simulink model "Reaching"  (R2024b)
settings: Solver=FixedStepDiscrete  StartTime=0.0  StopTime=inf  FixedStep=0.001  RelTol=1e-3
undefined symbols (not defined in the file): get
libraries: vrlib x3, PhanTorque_3Dof_Library_64Bits x1
settings Model: Creator=carlos.aldana  LastModifiedBy=alvinisac
settings SolverCC: AlgebraicLoopSolver=TrustRegion
settings DataIOCC: LimitDataPoints=on  SaveFormat=Array  ReturnWorkspaceOutputs=off
settings OptimizationCC: BlockReduction=off  BooleanDataType=off  LifeSpan=inf
settings DebuggingCC: SaveWithParameterizedLinksMsg=none  UnderspecifiedInitializationDetection=Classic  MergeDetectMultiDrivingBlocksExec=none  SignalResolutionControl=TryResolveAllWithWarning  UnconnectedInputMsg=warning  UnconnectedOutputMsg=warning  UnconnectedLineMsg=warning  AllowSymbolicDim=off  SFUnexpectedBacktrackingDiag=warning  SFNoUnconditionalDefaultTransitionDiag=warning  SFExecutionAtInitializationDiag=none  ArithmeticOperatorsInVariantConditions=warning
settings HardwareCC: ProdBitPerPointer=32  ProdBitPerSizeT=32  ProdBitPerPtrDiffT=32  ProdLargestAtomicFloat=None  ProdIntDivRoundTo=Undefined  ProdEndianess=Unspecified  ProdWordSize=32  ProdHWDeviceType=32-bit Generic  TargetUnknown=on
settings ModelReferenceCC: EnableRefExpFcnMdlSchedulingChecks=on  PropagateSignalLabelsOutOfModel=off
settings SFSimCC: SimUseLocalCustomCode=off  CustomCodeUndefinedFunction=UseInterfaceOnly
settings RTWCC: RTWUseLocalCustomCode=off  GPUComputeCapability=3.5  DLArmComputeVersion=19.05
settings CodeAppCC: StateflowObjectComments=on
settings GRTTargetCC: TargetLangStandard=C89/C90 (ANSI)
settings ConfigComp: CovMetricSettings=dw  CovSaveCumulativeToWorkspaceVar=on  CovSaveSingleToWorkspaceVar=on  CovExternalEMLEnable=off  CovSFcnEnable=off

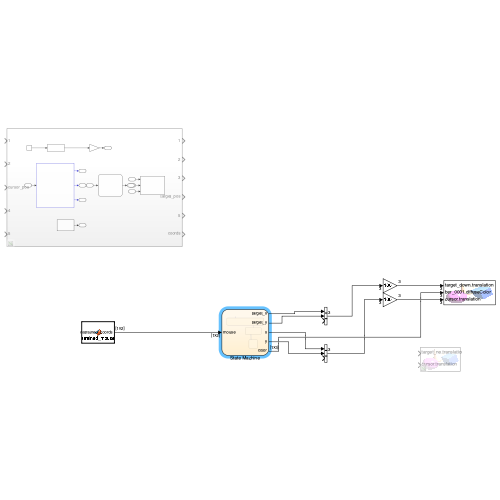
[thumbnail: Simulink's stored preview of the top-level diagram]
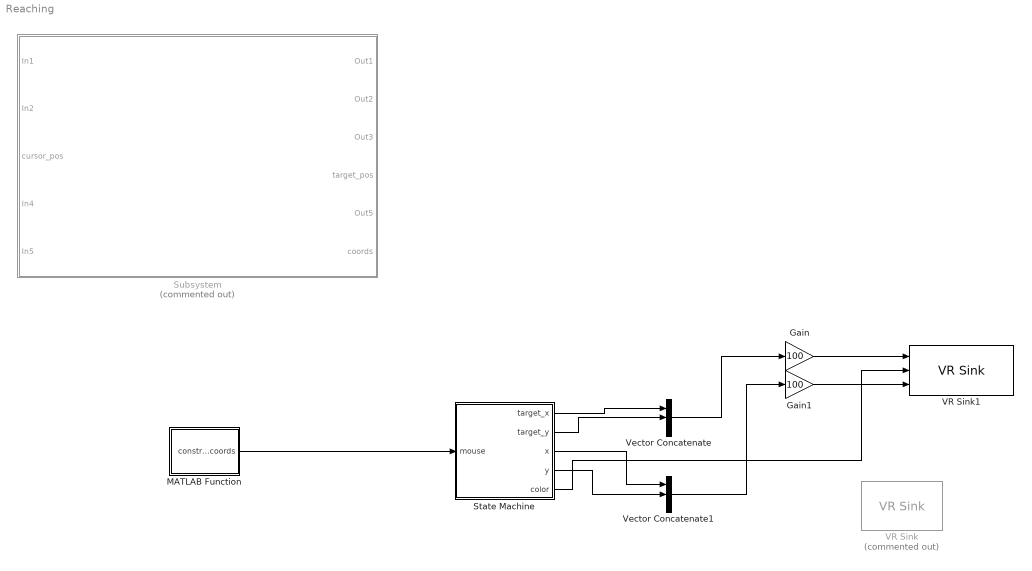
== system Reaching ==
  Gain : Gain  Gain=100
  Gain1 : Gain  Gain=100
  MATLAB Function : MATLAB Function  TreatAsAtomicUnit=on
  State Machine : Stateflow chart  TreatAsAtomicUnit=on
  Subsystem : Subsystem  Commented=on
  VR Sink : vrlib/VR Sink  Commented=on  InstantiateOnLoad=on  SampleTime=0.1  ViewEnable=on  RemoteChange=off  RemoteView=off  FieldsWritten=target_ne.translation.3.1.1.double#cursor.translation.3.1.1.double  WorldFileName=8_palline_color.wrl  AutoView=off  VideoDimensions=[]  AllowVariableSize=off
  VR Sink1 : vrlib/VR Sink  InstantiateOnLoad=on  SampleTime=0.1  ViewEnable=on  RemoteChange=off  RemoteView=off  FieldsWritten=target_down.translation.3.1.1.double#ber_0001.diffuseColor.3.1.1.double#cursor.translation.3.1.1.double  WorldFileName=VR_centerAndTarget.wrl  AutoView=off  VideoDimensions=[]  AllowVariableSize=off  FigureProperties="{'Position', 'Name', 'Viewpoint', 'CameraBound', 'CameraDirection', 'CameraPosition', 'CameraUpVector', 'ZoomFactor', 'Antialiasing', 'Headlight', 'Lighting', 'Sound', 'StatusBar', 'Stereo3D', 'Stereo3DCameraOffset', 'Stereo3DHIT', 'ToolBar', 'Textures', 'Transparency', 'Triad', 'Wireframe', 'NavZones', 'NavMode', 'NavSpeed', 'CaptureFileFormat', 'CaptureFileName', 'Record2DCompressMethod', 'Record2DCompressQuality', 'Record2D', 'Record2DFileName', 'Record2DFPS', 'NavPanel'; [5.0000000000000000e+00   1.0300000000000000e+02   5.7600000000000000e+02   3.5000000000000000e+02], '', '_untitled_1', 'on', [0.0000000000000000e+00   0.0000000000000000e+00  -1.0000000000000000e+00], [0.0000000000000000e+00   0.0000000000000000e+00   0.0000000000000000e+00], [0.0000000000000000e+00   1.0000000000000000e+00   0.0000000000000000e+00], [1.0000000000000000e+00], 'on', 'on', 'on', 'on', 'on', 'off', [1.0000000149011612e-01], [0.0000000000000000e+00], 'on', 'on', 'on', 'none', 'off', 'off', 'fly', 'normal', 'tif', '%f_anim_%n.tif', 'auto', [7.5000000000000000e+01], 'off', '%f_anim_%n.avi', 'auto', 'halfbar'}"
  Vector Concatenate : Concatenate  NumInputs=3
  Vector Concatenate1 : Concatenate  NumInputs=3
  wires:
  MATLAB Function/1(constrained_coords) -> State Machine/1(mouse)
  State Machine/1(target_x) -> Vector Concatenate/1
  State Machine/2(target_y) -> Vector Concatenate/2
  State Machine/4(y) -> Vector Concatenate1/2
  State Machine/3(x) -> Vector Concatenate1/1
  Vector Concatenate1/1 -> Gain1/1
  Vector Concatenate/1 -> Gain/1
  Gain/1 -> VR Sink1/1
  Gain1/1 -> VR Sink1/3
  State Machine/5(color) -> VR Sink1/2

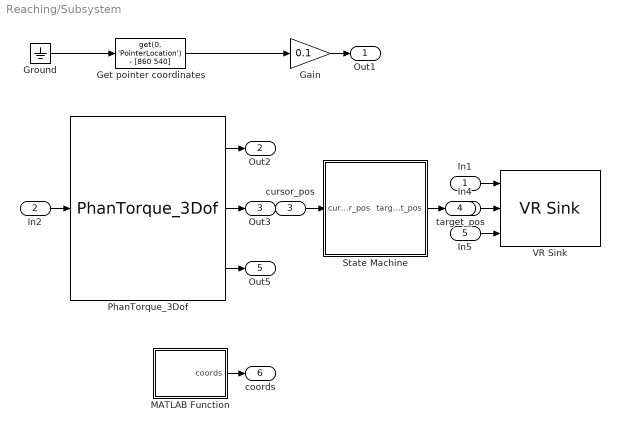
== system Reaching/Subsystem ==
  In1 : Inport
  In2 : Inport  Port=2
  cursor_pos : Inport  Port=3
  In4 : Inport  Port=4
  In5 : Inport  Port=5
  Gain : Gain  Gain=0.1
  Get pointer coordinates : MATLABFcn  MATLABFcn=get(0, 'PointerLocation') - [860 540]  OutputDimensions=2
  Ground : Ground
  MATLAB Function : MATLAB Function  TreatAsAtomicUnit=on
  PhanTorque_3Dof : PhanTorque_3Dof_Library_64Bits/PhanTorque_3Dof  Haptic_Name='Default Device'
  State Machine : Stateflow chart  TreatAsAtomicUnit=on
  VR Sink : vrlib/VR Sink  InstantiateOnLoad=on  SampleTime=0.1  ViewEnable=on  RemoteChange=off  RemoteView=off  FieldsWritten=target_down.translation.3.1.1.double#ber_0001.diffuseColor.3.1.1.double#cursor.translation.3.1.1.double  WorldFileName=VR_centerAndTarget.wrl  AutoView=off  VideoDimensions=[]  AllowVariableSize=off
  Out1 : Outport
  Out2 : Outport  Port=2
  Out3 : Outport  Port=3
  target_pos : Outport  Port=4
  Out5 : Outport  Port=5
  coords : Outport  Port=6
  wires:
  In5/1 -> VR Sink/3
  State Machine/1(target_pos) -> target_pos/1
  PhanTorque_3Dof/2 -> Out3/1
  PhanTorque_3Dof/3 -> Out5/1
  PhanTorque_3Dof/1 -> Out2/1
  cursor_pos/1 -> State Machine/1(cursor_pos)
  In4/1 -> VR Sink/2
  In2/1 -> PhanTorque_3Dof/1
  Get pointer coordinates/1 -> Gain/1
  MATLAB Function/1(coords) -> coords/1
  In1/1 -> VR Sink/1
  Gain/1 -> Out1/1
  Ground/1 -> Get pointer coordinates/1

== stateflow chart Reaching/Subsystem/State Machine ==
  state Initializing
    entry:
    counter =
    time =
    color = [0 1 1];
    radius = 10;
  state New_target
    entry:
  state Finish
  (default) -> Initializing
  New_target -> Finish
  data: cursor_pos input; target_pos output; counter local; time local; target_color local; radius local; angle local

== matlab function Reaching/Subsystem/MATLAB Function ==
  data: coords output
function coords = get_pointer_coordinates
    coords = get(0, 'PointerLocation');

== stateflow chart Reaching/State Machine ==
  state Initializing
    entry:
    four_target = [0 0.1; 0 -0.1; 0.1 0; -0.1 0; 0.07071 0.07071; 0.07071 -0.07071; -0.07071 0.07071; -0.07071 -0.07071];
  state New_target
    entry:
    target_x = four_target(n, 1);
    target_y = four_target(n, 2);
    %color = [0 1 0];
  state wait_2_sec1
    entry:
    color = [1 0 0]
  state Home_block
    entry:
    color = [0 1 0]
    x = mouse(1);
    y = mouse(2);
    target_x = 0;
    target_y = 0;
    err_x = abs(target_x - x);
    err_y = abs(target_y - y);
    during:
    x = mouse(1);
    y = mouse(2);
    err_x = abs(target_x - x);
    err_y = abs(target_y - y);
    %color = [1 0 0];
  state checker_block
    entry:
    color = [0 1 0];
    x = mouse(1);
    y = mouse(2);
    err_x = abs(target_x - x);
    err_y = abs(target_y - y);
    during:
    x = mouse(1);
    y = mouse(2);
    err_x = abs(target_x - x);
    err_y = abs(target_y - y);
    exit:
    color=[0 1 0];
  state wait_2_sec
    entry:
    color = [1 0 0]
  (default) -> Initializing
  Initializing -> New_target : {n=1;}
  wait_2_sec1 -> New_target : [after(1,sec)]
  Home_block -> wait_2_sec1 : [(err_x < 0.01 & err_y < 0.01) ]{n = n + 1; color = [1 0 0];}
  New_target -> checker_block
  checker_block -> wait_2_sec : [(err_x < 0.01 & err_y < 0.01) ]
  wait_2_sec -> Home_block : [after(1,sec)]
  data: target_x output; mouse input; err_x local; err_y local; four_target local; n local; target_y output; x output; y output; color output

== matlab function Reaching/MATLAB Function ==
  data: constrained_coords output
function constrained_coords = get_constrained_mouse_coords()
    % Declare 'get' as extrinsic to run in MATLAB workspace
    coder.extrinsic('get');
    
    % Initialize output to avoid size/type mismatch
    constrained_coords = [0.0, 0.0]; % Initialize as a [1x2] double vector

    % Call the extrinsic function to get pointer location
    pointer_coords = [0, 0]; % Initialize to avoid simulation issues
    pointer_coords = get(0, 'PointerLocation');

    % Cast mxArray output to double to ensure compatibility
    pointer_coords = double(pointer_coords);

    % Scale pointer coordinates to normalized values (example: [-0.1, 0.1])
    screen_width = 1440;  % Replace with your screen width or x - axis
    screen_height = 900; % Replace with your screen height or Y - axis

    % Normalize to [-1, 1]
    x_norm = (pointer_coords(1) - screen_width / 2) / (screen_width / 2);
    y_norm = (pointer_coords(2) - screen_height / 2) / (screen_height / 2);

    % Scale to [-0.1, 0.1] range
    x_scaled = x_norm * 0.1;
    y_scaled = y_norm * 0.1;

    % Constrain to [-0.1, 0.1]
    constrained_x = max(-0.1, min(0.1, x_scaled));
    constrained_y = max(-0.1, min(0.1, y_scaled));

    % Output constrained coordinates
    constrained_coords = [constrained_x, constrained_y];
end
